simulink model "modBPSKsurporteuse"  (Simulink 10.1)
settings: Solver=FixedStepDiscrete  StartTime=0.0  StopTime=10  RelTol=1e-3
libraries: commutil2 x5, dspsrcs4 x4, dspsigops x4, commrandsrc3 x2
settings Model: LogicAnalyzerSignalOrdering=70be029a-c879-49fd-8142-2062ffae8c01,78a88755-5817-4797-a273-ee478a7c3c2d,9a052def-c5fe-4504-a556-fa7b767558ac,8554bb34-e2ba-4d5f-bec6-1929df8b304a,67ea8bbd-5709-4836-9b08-5aa86dc41909,40e969c7-c572-493e-8027-6861ae4e2639,31c4ce99-13f9-42fa-8fab-d4a79b2f203f,65ba6bbf-b89b-449c-b974-0b0e4ba483cd,8c77df25-ac90-4703-b197-bb0c03b5bdee,58304572-a802-46ce-ba81-d601c7bc0847,879bd828-2ac7-4caa-94ef-6949ebba491e,821e6c2c-d359-4312-84e1-6ac9f0da9194,0f964614-90d7-4bd4-afc6-7c8d85a44781,15d3bc02-27ed-47cc-8223-1bb63c847540,216596cd-ea4a-4e30-a72e-4aff735e22aa,250f0ea8-c39a-49f7-863f-c86bb904ed06,e83e8e0a-d250-4af6-bb48-efc28f5c8d7c,5828b797-5f98-4ab5-bd12-89e809ab75dc,3fdc4b80-71cd-4be3-be3c-e5d3c8a346cc,ff8d1946-f4bd-4671-ac48-3eb882c5c483  Creator=iba  LastModifiedBy=iba
settings DataIOCC: SaveFormat=Dataset  ReturnWorkspaceOutputs=on
settings OptimizationCC: LifeSpan=auto
settings DebuggingCC: UnderspecifiedInitializationDetection=Simplified  MergeDetectMultiDrivingBlocksExec=error  SFUnexpectedBacktrackingDiag=error  SFNoUnconditionalDefaultTransitionDiag=error  SFExecutionAtInitializationDiag=warning  ArithmeticOperatorsInVariantConditions=error
settings HardwareCC: ProdBitPerPointer=64  ProdBitPerSizeT=64  ProdBitPerPtrDiffT=64  ProdLargestAtomicFloat=Float  ProdIntDivRoundTo=Zero  ProdEndianess=LittleEndian  ProdWordSize=64  ProdHWDeviceType=Intel->x86-64 (Windows64)
settings ModelReferenceCC: PropagateSignalLabelsOutOfModel=on
settings SFSimCC: SimUseLocalCustomCode=on  CustomCodeUndefinedFunction=FilterOut
settings RTWCC: RTWUseLocalCustomCode=on
settings CodeAppCC: StateflowObjectComments=off
settings GRTTargetCC: TargetLangStandard=C99 (ISO)  CombineOutputUpdateFcns=on  GRTInterface=off
settings ConfigComp: CovMetricSettings=dwe  CovHtmlReporting=off  CovSaveCumulativeToWorkspaceVar=off  CovSaveSingleToWorkspaceVar=off  CovExternalEMLEnable=on

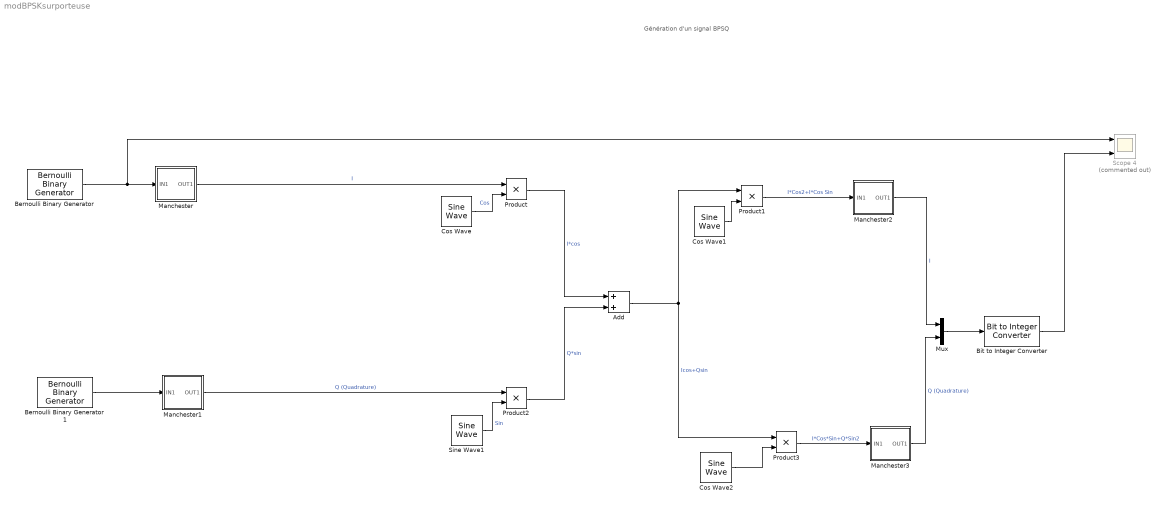
== system modBPSKsurporteuse ==
  note: Génération d'un signal BPSQ
  Add : Sum
  "Bernoulli Binary Generator " : commrandsrc3/Bernoulli Binary Generator  ProbabilityOfZero=0.5  SeedSource=Parameter  Seed=61  SampleTime=1  SamplesPerFrame=1  OutputDataType=double  SimulateUsing=Interpreted execution
  Bernoulli Binary Generator 1 : commrandsrc3/Bernoulli Binary Generator  ProbabilityOfZero=0.5  SeedSource=Parameter  Seed=61  SampleTime=1  SamplesPerFrame=1  OutputDataType=double  SimulateUsing=Interpreted execution
  Bit to Integer Converter : commutil2/Bit to Integer Converter  nbits=2  bitOrder=MSB first  signedOutputValues=Unsigned  outDtype=uint32  outDtypeSigned=Inherit via internal rule
  Cos Wave : dspsrcs4/Sine Wave  Amplitude=1  Frequency=5  Phase=pi/2  SampleMode=Discrete  OutComplex=Real  CompMethod=Trigonometric fcn  TableSize=Speed  SampleTime=1/100  SamplesPerFrame=1  ResetState=Restart at time zero  OutputFrames=off  dataType=double  wordLen=16  udDataType=sfix(16)  fracBitsMode=Best precision  numFracBits=15  OutDataTypeStr=double  LastOutDataTypeStr=double
  Cos Wave1 : dspsrcs4/Sine Wave  Amplitude=1  Frequency=5  Phase=pi/2  SampleMode=Discrete  OutComplex=Real  CompMethod=Trigonometric fcn  TableSize=Speed  SampleTime=1/100  SamplesPerFrame=1  ResetState=Restart at time zero  OutputFrames=off  dataType=double  wordLen=16  udDataType=sfix(16)  fracBitsMode=Best precision  numFracBits=15  OutDataTypeStr=double  LastOutDataTypeStr=double
  Cos Wave2 : dspsrcs4/Sine Wave  Amplitude=1  Frequency=5  Phase=0  SampleMode=Discrete  OutComplex=Real  CompMethod=Trigonometric fcn  TableSize=Speed  SampleTime=1/100  SamplesPerFrame=1  ResetState=Restart at time zero  OutputFrames=off  dataType=double  wordLen=16  udDataType=sfix(16)  fracBitsMode=Best precision  numFracBits=15  OutDataTypeStr=double  LastOutDataTypeStr=double
  Manchester : Subsystem
  Manchester1 : Subsystem
  Manchester2 : Subsystem
  Manchester3 : Subsystem
  Mux : Mux  Inputs=2
  Product{,1..3} (4 alike) : Product
  Scope 4 : Scope  Commented=on  NumInputPorts=3
  Sine Wave1 : dspsrcs4/Sine Wave  Amplitude=1  Frequency=5  Phase=0  SampleMode=Discrete  OutComplex=Real  CompMethod=Trigonometric fcn  TableSize=Speed  SampleTime=1/100  SamplesPerFrame=1  ResetState=Restart at time zero  OutputFrames=off  dataType=double  wordLen=16  udDataType=sfix(16)  fracBitsMode=Best precision  numFracBits=15  OutDataTypeStr=double  LastOutDataTypeStr=double
  wires:
  Cos Wave/1 -> Product/2  "Cos"
  Cos Wave1/1 -> Product1/2
  "Bernoulli Binary Generator "/1 -> Scope 4/1, Manchester/1(IN1)
  Sine Wave1/1 -> Product2/2  "Sin"
  Cos Wave2/1 -> Product3/2
  Manchester1/1(OUT1) -> Product2/1  "Q (Quadrature)"
  Product/1 -> Add/1  "I*cos"
  Product2/1 -> Add/2  "Q*sin"
  Add/1 -> Product3/1, Product1/1  "Icos+Qsin"
  Bernoulli Binary Generator 1/1 -> Manchester1/1(IN1)
  Manchester/1(OUT1) -> Product/1  "I"
  Product3/1 -> Manchester3/1(IN1)  "I*Cos*Sin+Q*Sin2"
  Product1/1 -> Manchester2/1(IN1)  "I*Cos2+I*Cos Sin"
  Manchester2/1(OUT1) -> Mux/1  "I"
  Manchester3/1(OUT1) -> Mux/2  "Q (Quadrature)"
  Mux/1 -> Bit to Integer Converter/1
  Bit to Integer Converter/1 -> Scope 4/3

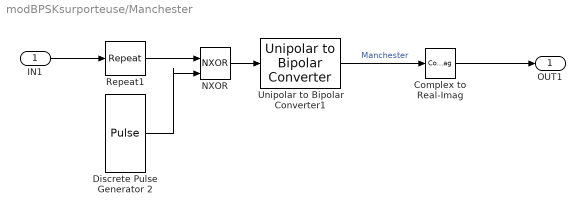
== system modBPSKsurporteuse/Manchester ==
  IN1 : Inport
  Complex to Real-Imag : ComplexToRealImag  Output=Real
  "Discrete Pulse Generator 2  " : DiscretePulseGenerator  SampleTime=0.01
  "NXOR " : Logic  Operator=NXOR  IconShape=distinctive  AllPortsSameDT=off  OutDataTypeStr=boolean
  Repeat1 : dspsigops/Repeat  N=2  InputProcessing=Columns as channels (frame based)  RateOptions=Enforce single-rate processing  ic=0  mode=Unused parameter value
  Unipolar to Bipolar Converter1 : commutil2/Unipolar to Bipolar Converter  M=2  polarity=Positive  dataType=double
  OUT1 : Outport
  wires:
  IN1/1 -> Repeat1/1
  "NXOR "/1 -> Unipolar to Bipolar Converter1/1
  "Discrete Pulse Generator 2  "/1 -> "NXOR "/2
  Repeat1/1 -> "NXOR "/1
  Unipolar to Bipolar Converter1/1 -> Complex to Real-Imag/1  "Manchester"
  Complex to Real-Imag/1 -> OUT1/1

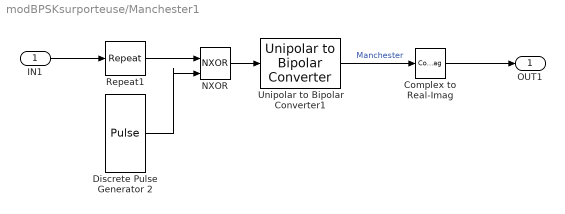
== system modBPSKsurporteuse/Manchester1 ==
  IN1 : Inport
  Complex to Real-Imag : ComplexToRealImag  Output=Imag
  "Discrete Pulse Generator 2  " : DiscretePulseGenerator  SampleTime=0.01
  "NXOR " : Logic  Operator=NXOR  IconShape=distinctive  AllPortsSameDT=off  OutDataTypeStr=boolean
  Repeat1 : dspsigops/Repeat  N=2  InputProcessing=Columns as channels (frame based)  RateOptions=Enforce single-rate processing  ic=0  mode=Unused parameter value
  Unipolar to Bipolar Converter1 : commutil2/Unipolar to Bipolar Converter  M=2  polarity=Positive  dataType=double
  OUT1 : Outport
  wires:
  IN1/1 -> Repeat1/1
  "NXOR "/1 -> Unipolar to Bipolar Converter1/1
  "Discrete Pulse Generator 2  "/1 -> "NXOR "/2
  Repeat1/1 -> "NXOR "/1
  Complex to Real-Imag/1 -> OUT1/1
  Unipolar to Bipolar Converter1/1 -> Complex to Real-Imag/1  "Manchester"

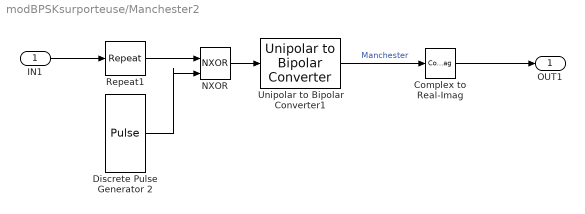
== system modBPSKsurporteuse/Manchester2 ==
  IN1 : Inport
  Complex to Real-Imag : ComplexToRealImag  Output=Real
  "Discrete Pulse Generator 2  " : DiscretePulseGenerator  SampleTime=0.01
  "NXOR " : Logic  Operator=NXOR  IconShape=distinctive  AllPortsSameDT=off  OutDataTypeStr=boolean
  Repeat1 : dspsigops/Repeat  N=2  InputProcessing=Columns as channels (frame based)  RateOptions=Enforce single-rate processing  ic=0  mode=Unused parameter value
  Unipolar to Bipolar Converter1 : commutil2/Unipolar to Bipolar Converter  M=2  polarity=Positive  dataType=double
  OUT1 : Outport
  wires:
  Complex to Real-Imag/1 -> OUT1/1
  Unipolar to Bipolar Converter1/1 -> Complex to Real-Imag/1  "Manchester"
  Repeat1/1 -> "NXOR "/1
  "Discrete Pulse Generator 2  "/1 -> "NXOR "/2
  "NXOR "/1 -> Unipolar to Bipolar Converter1/1
  IN1/1 -> Repeat1/1

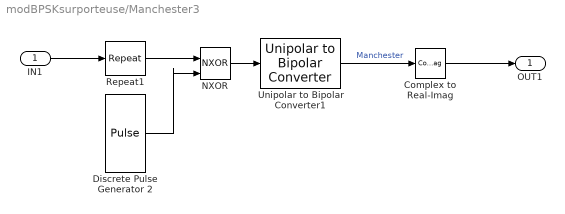
== system modBPSKsurporteuse/Manchester3 ==
  IN1 : Inport
  Complex to Real-Imag : ComplexToRealImag  Output=Imag
  "Discrete Pulse Generator 2  " : DiscretePulseGenerator  SampleTime=0.01
  "NXOR " : Logic  Operator=NXOR  IconShape=distinctive  AllPortsSameDT=off  OutDataTypeStr=boolean
  Repeat1 : dspsigops/Repeat  N=2  InputProcessing=Columns as channels (frame based)  RateOptions=Enforce single-rate processing  ic=0  mode=Unused parameter value
  Unipolar to Bipolar Converter1 : commutil2/Unipolar to Bipolar Converter  M=2  polarity=Positive  dataType=double
  OUT1 : Outport
  wires:
  Unipolar to Bipolar Converter1/1 -> Complex to Real-Imag/1  "Manchester"
  Complex to Real-Imag/1 -> OUT1/1
  Repeat1/1 -> "NXOR "/1
  "Discrete Pulse Generator 2  "/1 -> "NXOR "/2
  "NXOR "/1 -> Unipolar to Bipolar Converter1/1
  IN1/1 -> Repeat1/1
